simulink library "INT_EngSpd_DD"  (R2016b)
settings: Solver=VariableStepAuto  StartTime=0.0  StopTime=10.0  RelTol=1e-3
settings Model: Creator=yangyang  LastModifiedBy=yangyang

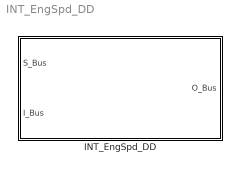
== system INT_EngSpd_DD ==
  INT_EngSpd_DD : Subsystem

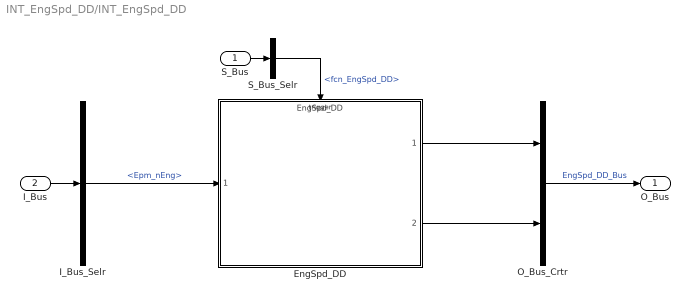
== system INT_EngSpd_DD/INT_EngSpd_DD ==
  S_Bus : Inport
  I_Bus : Inport  Port=2
  EngSpd_DD : ModelReference  ModelNameDialog=EngSpd_DD  SimulationMode=Normal  ModelReferenceVersion=1.23  TriggerPortName=function  TriggerPortTriggerType=function-call  TriggerPortStatesWhenEnabling=held
  I_Bus_Selr : BusSelector  OutputSignals=Epm_nEng
  O_Bus_Crtr : BusCreator  Inputs=2
  S_Bus_Selr : BusSelector  OutputSignals=fcn_EngSpd_DD
  O_Bus : Outport
  wires:
  S_Bus_Selr/1 -> EngSpd_DD/Trigger  "<fcn_EngSpd_DD>"
  S_Bus/1 -> S_Bus_Selr/1
  I_Bus/1 -> I_Bus_Selr/1
  I_Bus_Selr/1 -> EngSpd_DD/1  "<Epm_nEng>"
  O_Bus_Crtr/1 -> O_Bus/1  "EngSpd_DD_Bus"
  EngSpd_DD/1 -> O_Bus_Crtr/1
  EngSpd_DD/2 -> O_Bus_Crtr/2
